simulink model "TestFilter"  (R2022b)
settings: Solver=FixedStepAuto  StartTime=0.0  StopTime=T  FixedStep=dt  RelTol=1e-3
values from neighbouring files (symbols this model uses):
  Parameter = DefaultParameter_SLOW2DOF    [Exercise05_TowerDamperDesign.m]    (also in Exercise05_TowerDamperTestTurbulentWind.m = DefaultParameter_FBv1_ADv14(Parameter); Exercise05_TowerDamperTestWindStep.m = DefaultParameter_FBv1_ADv14(Parameter); Exercise06_PitchControllerDesign.m = DefaultParameter_FBv1_ADv14(Parameter); HowToFindRatedWindSpeed.m = DefaultParameter_FBv1_ADv14(Parameter))
undefined symbols (not defined in the file or in its folder): Gain, x2_t0
settings Model: Creator=felix  LastModifiedBy=felix

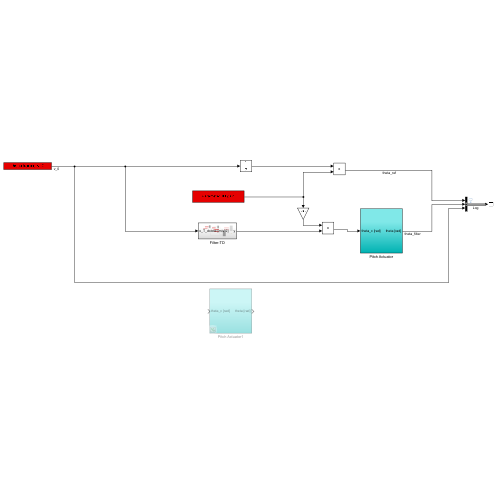
[thumbnail: Simulink's stored preview of the top-level diagram]
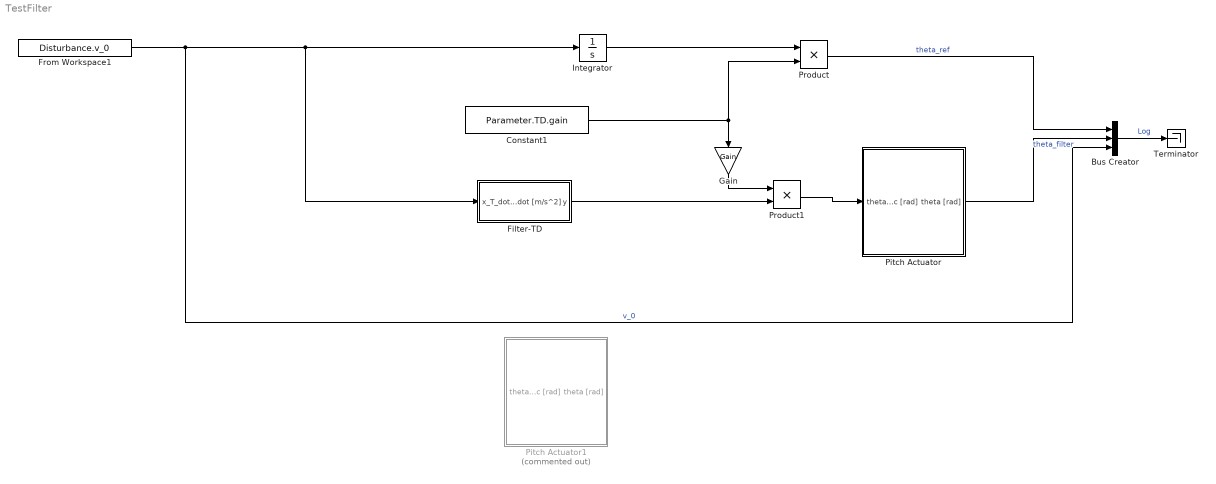
== system TestFilter ==
  Bus Creator : BusCreator  Inputs=3
  Constant1 : Constant  Value=Parameter.TD.gain
  Filter-TD : Subsystem
  From Workspace1 : FromWorkspace  VariableName=Disturbance.v_0
  Gain : Gain  Gain=Gain
  Integrator : Integrator
  Pitch Actuator : Subsystem
  Pitch Actuator1 : Subsystem  Commented=on
  Product : Product
  Product1 : Product
  Terminator : Terminator
  wires:
  From Workspace1/1 -> Bus Creator/3, Integrator/1, Filter-TD/1(x_T_dotdot [m/s^2])  "v_0"
  Integrator/1 -> Product/1
  Bus Creator/1 -> Terminator/1  "Log"
  Constant1/1 -> Gain/1, Product/2
  Product/1 -> Bus Creator/1  "theta_ref"
  Pitch Actuator/1(theta [rad]) -> Bus Creator/2  "theta_filter"
  Filter-TD/1(y) -> Product1/2
  Product1/1 -> Pitch Actuator/1(theta_c [rad])
  Gain/1 -> Product1/1

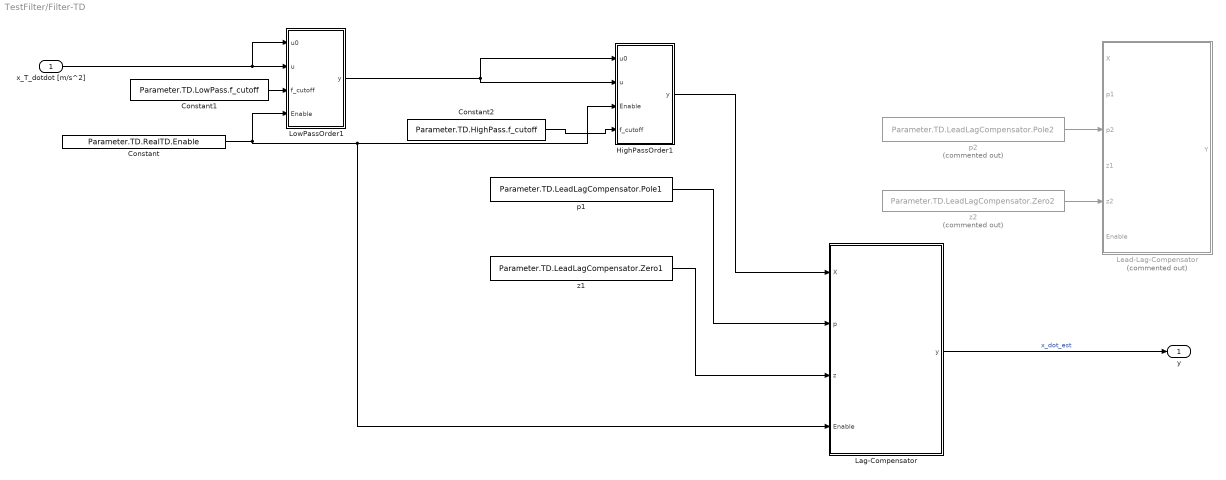
== system TestFilter/Filter-TD ==
  x_T_dotdot [m/s^2] : Inport
  Constant : Constant  Value=Parameter.TD.RealTD.Enable
  Constant1 : Constant  Value=Parameter.TD.LowPass.f_cutoff
  Constant2 : Constant  Value=Parameter.TD.HighPass.f_cutoff
  HighPassOrder1 : Subsystem
  Lag-Compensator : Subsystem
  Lead-Lag-Compensator : Subsystem  Commented=on
  LowPassOrder1 : Subsystem
  p1 : Constant  Value=Parameter.TD.LeadLagCompensator.Pole1
  p2 : Constant  Commented=on  Value=Parameter.TD.LeadLagCompensator.Pole2
  z1 : Constant  Value=Parameter.TD.LeadLagCompensator.Zero1
  z2 : Constant  Commented=on  Value=Parameter.TD.LeadLagCompensator.Zero2
  y : Outport
  wires:
  Constant/1 -> Lag-Compensator/4(Enable), HighPassOrder1/3(Enable), LowPassOrder1/4(Enable)
  Constant1/1 -> LowPassOrder1/3(f_cutoff)
  Constant2/1 -> HighPassOrder1/4(f_cutoff)
  LowPassOrder1/1(y) -> HighPassOrder1/1(u0), HighPassOrder1/2(u)
  x_T_dotdot [m/s^2]/1 -> LowPassOrder1/1(u0), LowPassOrder1/2(u)
  HighPassOrder1/1(y) -> Lag-Compensator/1(X)
  p1/1 -> Lag-Compensator/2(p)
  z1/1 -> Lag-Compensator/3(z)
  Lag-Compensator/1(y) -> y/1  "x_dot_est"
  z2/1 -> Lead-Lag-Compensator/5(z2)
  p2/1 -> Lead-Lag-Compensator/3(p2)

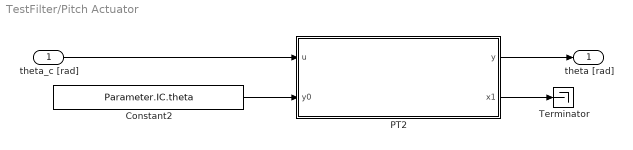
== system TestFilter/Pitch Actuator ==
  theta_c [rad] : Inport
  Constant2 : Constant  Value=Parameter.IC.theta
  PT2 : Subsystem  mask{omega=Parameter.PitchActuator.omega, xi=Parameter.PitchActuator.xi, x1_max=Parameter.PitchActuator.theta_dot_max, x1_min=-Parameter.PitchActuator.theta_dot_max, x2_max=Parameter.PitchActuator.theta_max, x2_min=Parameter.PitchActuator.theta_min}
      mask prompts: omega "undamped natural frequency [rad/s]"; xi "damping factor [-]"; x1_max "Upper bound x1"; x1_min "Lower bound x1"; x2_max "Upper bound x2"; x2_min "Lower bound x2"
      mask Display:
      | disp(['omega = ',num2str(omega),'\n'...
      |     ,'xi = ',num2str(xi)])
      | port_label('output',1,'y')
      | port_label('output',2,'x1')
      | port_label('input',2,'y0')
      | port_label('input',1,'u')
  Terminator : Terminator
  theta [rad] : Outport
  wires:
  theta_c [rad]/1 -> PT2/1(u)
  Constant2/1 -> PT2/2(y0)
  PT2/1(y) -> theta [rad]/1
  PT2/2(x1) -> Terminator/1

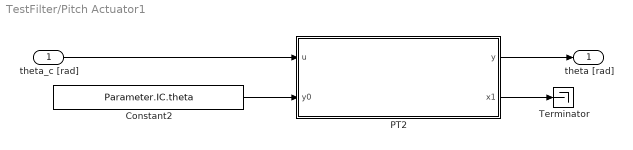
== system TestFilter/Pitch Actuator1 ==
  theta_c [rad] : Inport
  Constant2 : Constant  Value=Parameter.IC.theta
  PT2 : Subsystem  mask{omega=Parameter.PitchActuator.omega, xi=Parameter.PitchActuator.xi, x1_max=Parameter.PitchActuator.theta_dot_max, x1_min=-Parameter.PitchActuator.theta_dot_max, x2_max=Parameter.PitchActuator.theta_max, x2_min=Parameter.PitchActuator.theta_min}
      mask prompts: omega "undamped natural frequency [rad/s]"; xi "damping factor [-]"; x1_max "Upper bound x1"; x1_min "Lower bound x1"; x2_max "Upper bound x2"; x2_min "Lower bound x2"
      mask Display:
      | disp(['omega = ',num2str(omega),'\n'...
      |     ,'xi = ',num2str(xi)])
      | port_label('output',1,'y')
      | port_label('output',2,'x1')
      | port_label('input',2,'y0')
      | port_label('input',1,'u')
  Terminator : Terminator
  theta [rad] : Outport
  wires:
  theta_c [rad]/1 -> PT2/1(u)
  Constant2/1 -> PT2/2(y0)
  PT2/1(y) -> theta [rad]/1
  PT2/2(x1) -> Terminator/1

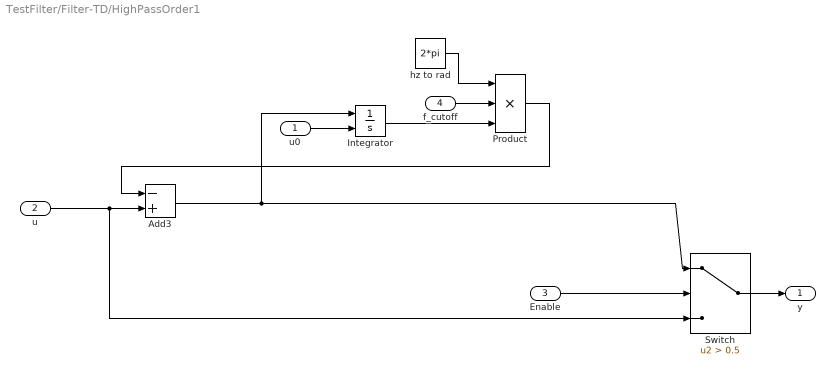
== system TestFilter/Filter-TD/HighPassOrder1 ==
  u0 : Inport
  u : Inport  Port=2
  Enable : Inport  Port=3
  f_cutoff : Inport  Port=4
  Add3 : Sum  Inputs=-+
  Integrator : Integrator  InitialConditionSource=external
  Product : Product  Inputs=3  RndMeth=Zero
  Switch : Switch  Criteria=u2 > Threshold  Threshold=0.5  SaturateOnIntegerOverflow=off  InputSameDT=off
  hz to rad : Constant  Value=2*pi
  y : Outport  VectorParamsAs1DForOutWhenUnconnected=off
  wires:
  Switch/1 -> y/1
  Enable/1 -> Switch/2
  u/1 -> Add3/2, Switch/3
  hz to rad/1 -> Product/1
  Add3/1 -> Integrator/1, Switch/1
  Integrator/1 -> Product/3
  Product/1 -> Add3/1
  u0/1 -> Integrator/2
  f_cutoff/1 -> Product/2

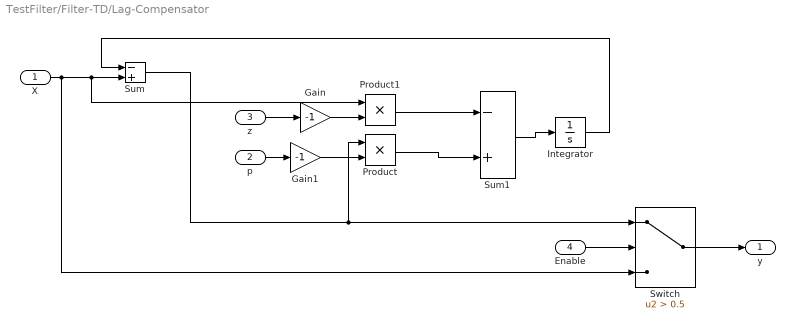
== system TestFilter/Filter-TD/Lag-Compensator ==
  X : Inport
  p : Inport  Port=2
  z : Inport  Port=3
  Enable : Inport  Port=4
  Gain : Gain  Gain=-1
  Gain1 : Gain  Gain=-1
  Integrator : Integrator
  Product : Product
  Product1 : Product
  Sum : Sum  Inputs=-+
  Sum1 : Sum  Inputs=-+
  Switch : Switch  Criteria=u2 > Threshold  Threshold=0.5  SaturateOnIntegerOverflow=off  InputSameDT=off
  y : Outport
  wires:
  X/1 -> Switch/3, Product1/1, Sum/2
  z/1 -> Gain/1
  p/1 -> Gain1/1
  Switch/1 -> y/1
  Sum/1 -> Product/1, Switch/1
  Product/1 -> Sum1/2
  Product1/1 -> Sum1/1
  Sum1/1 -> Integrator/1
  Integrator/1 -> Sum/1
  Enable/1 -> Switch/2
  Gain1/1 -> Product/2
  Gain/1 -> Product1/2

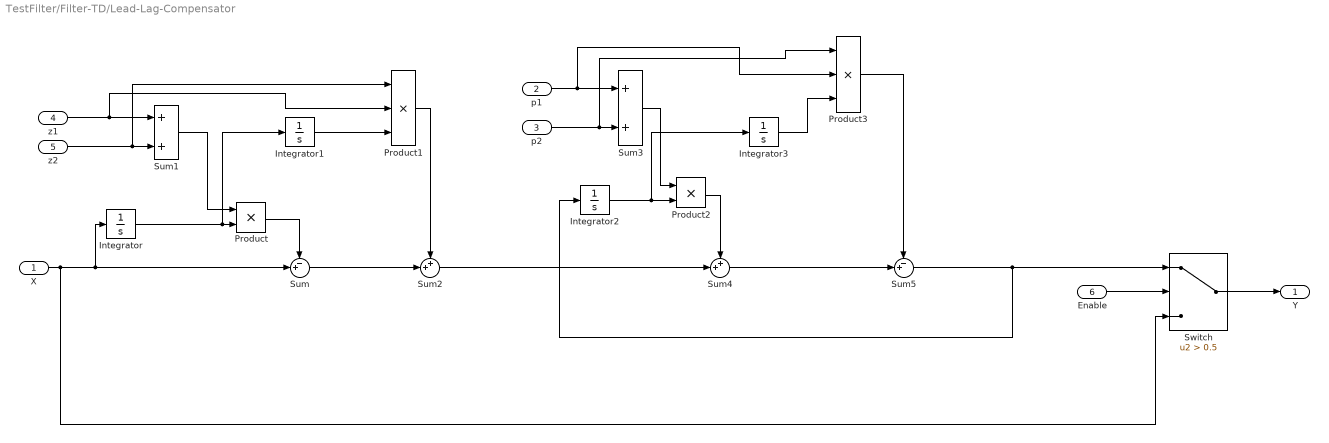
== system TestFilter/Filter-TD/Lead-Lag-Compensator ==
  X : Inport
  p1 : Inport  Port=2
  p2 : Inport  Port=3
  z1 : Inport  Port=4
  z2 : Inport  Port=5
  Enable : Inport  Port=6
  Integrator{,1..3} (4 alike) : Integrator
  Product : Product
  Product1 : Product  Inputs=3
  Product2 : Product
  Product3 : Product  Inputs=3
  Sum : Sum  Inputs=-+|
  Sum1 : Sum
  Sum2 : Sum  Inputs=++|
  Sum3 : Sum
  Sum4 : Sum  Inputs=++|
  Sum5 : Sum  Inputs=-+|
  Switch : Switch  Criteria=u2 > Threshold  Threshold=0.5  SaturateOnIntegerOverflow=off  InputSameDT=off
  Y : Outport
  wires:
  X/1 -> Switch/3, Integrator/1, Sum/2
  z1/1 -> Product1/2, Sum1/1
  z2/1 -> Product1/1, Sum1/2
  Integrator/1 -> Integrator1/1, Product/2
  Sum1/1 -> Product/1
  Product/1 -> Sum/1
  Integrator1/1 -> Product1/3
  Sum/1 -> Sum2/2
  Product1/1 -> Sum2/1
  p1/1 -> Product3/2, Sum3/1
  p2/1 -> Product3/1, Sum3/2
  Sum2/1 -> Sum4/2
  Sum3/1 -> Product2/1
  Sum4/1 -> Sum5/2
  Sum5/1 -> Switch/1, Integrator2/1
  Integrator2/1 -> Integrator3/1, Product2/2
  Product2/1 -> Sum4/1
  Integrator3/1 -> Product3/3
  Product3/1 -> Sum5/1
  Switch/1 -> Y/1
  Enable/1 -> Switch/2

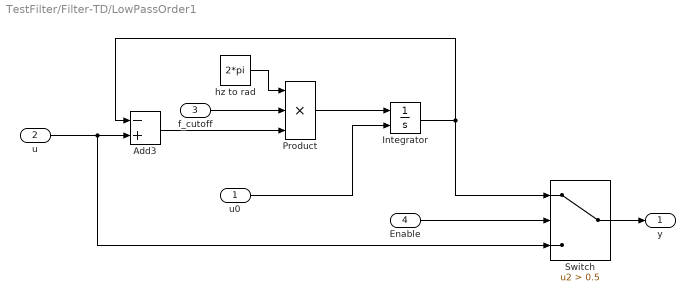
== system TestFilter/Filter-TD/LowPassOrder1 ==
  u0 : Inport
  u : Inport  Port=2
  f_cutoff : Inport  Port=3
  Enable : Inport  Port=4
  Add3 : Sum  Inputs=-+
  Integrator : Integrator  InitialConditionSource=external
  Product : Product  Inputs=3  RndMeth=Zero
  Switch : Switch  Criteria=u2 > Threshold  Threshold=0.5  SaturateOnIntegerOverflow=off  InputSameDT=off
  hz to rad : Constant  Value=2*pi
  y : Outport  VectorParamsAs1DForOutWhenUnconnected=off
  wires:
  u0/1 -> Integrator/2
  Switch/1 -> y/1
  Enable/1 -> Switch/2
  u/1 -> Add3/2, Switch/3
  Integrator/1 -> Switch/1, Add3/1
  Product/1 -> Integrator/1
  Add3/1 -> Product/3
  f_cutoff/1 -> Product/2
  hz to rad/1 -> Product/1

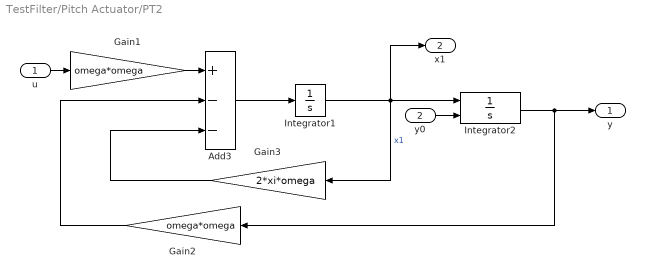
== system TestFilter/Pitch Actuator/PT2 ==
  u : Inport
  y0 : Inport  Port=2
  Add3 : Sum  Inputs=+--
  Gain1 : Gain  Gain=omega*omega  SaturateOnIntegerOverflow=on  OutDataTypeStr=Inherit: Same as input  ParamDataTypeStr=Inherit: Same as input
  Gain2 : Gain  Gain=omega*omega  SaturateOnIntegerOverflow=on  OutDataTypeStr=Inherit: Same as input  ParamDataTypeStr=Inherit: Same as input
  Gain3 : Gain  Gain=2*xi*omega  SaturateOnIntegerOverflow=on  OutDataTypeStr=Inherit: Same as input  ParamDataTypeStr=Inherit: Same as input
  Integrator1 : Integrator  UpperSaturationLimit=x1_max  LowerSaturationLimit=x1_min
  Integrator2 : Integrator  InitialConditionSource=external  InitialCondition=x2_t0  UpperSaturationLimit=x2_max  LowerSaturationLimit=x2_min
  y : Outport
  x1 : Outport  Port=2
  wires:
  Gain3/1 -> Add3/3
  u/1 -> Gain1/1
  Add3/1 -> Integrator1/1
  Gain1/1 -> Add3/1
  Gain2/1 -> Add3/2
  Integrator1/1 -> x1/1, Gain3/1, Integrator2/1  "x1"
  y0/1 -> Integrator2/2
  Integrator2/1 -> Gain2/1, y/1

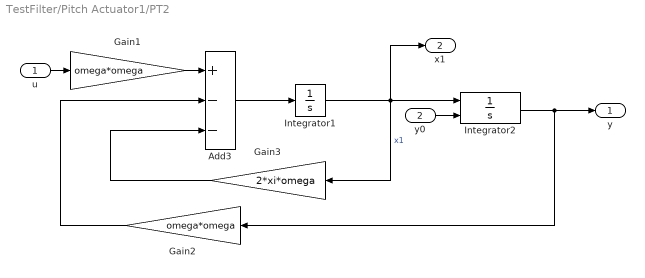
== system TestFilter/Pitch Actuator1/PT2 ==
  u : Inport
  y0 : Inport  Port=2
  Add3 : Sum  Inputs=+--
  Gain1 : Gain  Gain=omega*omega  SaturateOnIntegerOverflow=on  OutDataTypeStr=Inherit: Same as input  ParamDataTypeStr=Inherit: Same as input
  Gain2 : Gain  Gain=omega*omega  SaturateOnIntegerOverflow=on  OutDataTypeStr=Inherit: Same as input  ParamDataTypeStr=Inherit: Same as input
  Gain3 : Gain  Gain=2*xi*omega  SaturateOnIntegerOverflow=on  OutDataTypeStr=Inherit: Same as input  ParamDataTypeStr=Inherit: Same as input
  Integrator1 : Integrator  LimitOutput=on  UpperSaturationLimit=x1_max  LowerSaturationLimit=x1_min
  Integrator2 : Integrator  InitialConditionSource=external  InitialCondition=x2_t0  LimitOutput=on  UpperSaturationLimit=x2_max  LowerSaturationLimit=x2_min
  y : Outport
  x1 : Outport  Port=2
  wires:
  Gain3/1 -> Add3/3
  u/1 -> Gain1/1
  Add3/1 -> Integrator1/1
  Gain1/1 -> Add3/1
  Gain2/1 -> Add3/2
  Integrator1/1 -> x1/1, Gain3/1, Integrator2/1  "x1"
  y0/1 -> Integrator2/2
  Integrator2/1 -> Gain2/1, y/1
